simulink model "GCS"  (R2023a)
settings: Solver=FixedStepAuto  StartTime=0.0  StopTime=inf  FixedStep=1/100  RelTol=1e-3
undefined symbols (not defined in the file or in its folder): ARMED, AUX1, AUX2, f, MODE, NULL, Payload, Pitch, Roll, Throttle, Yaw
libraries: uavmavlinklib x3, vrlib x3, instrumentlib x2, instrumentseriallib x2, slrealtimeiplib x2, aerolibanimutils x1
settings Model: Creator=amc0121  LastModifiedBy=thesa
settings DebuggingCC: UnconnectedInputMsg=warning  UnconnectedOutputMsg=warning  UnconnectedLineMsg=warning
settings ModelReferenceCC: EnableRefExpFcnMdlSchedulingChecks=on
settings RTWCC: DLArmComputeVersion=19.05

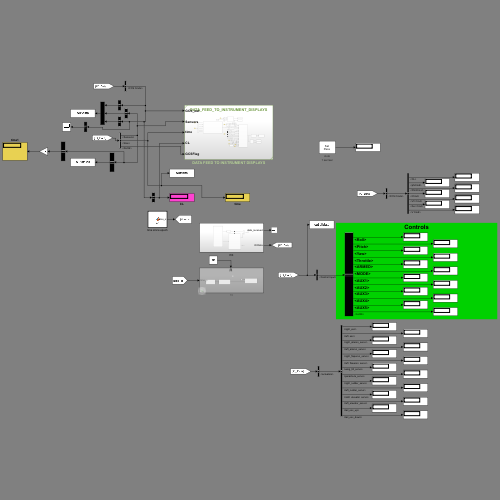
[thumbnail: Simulink's stored preview of the top-level diagram]
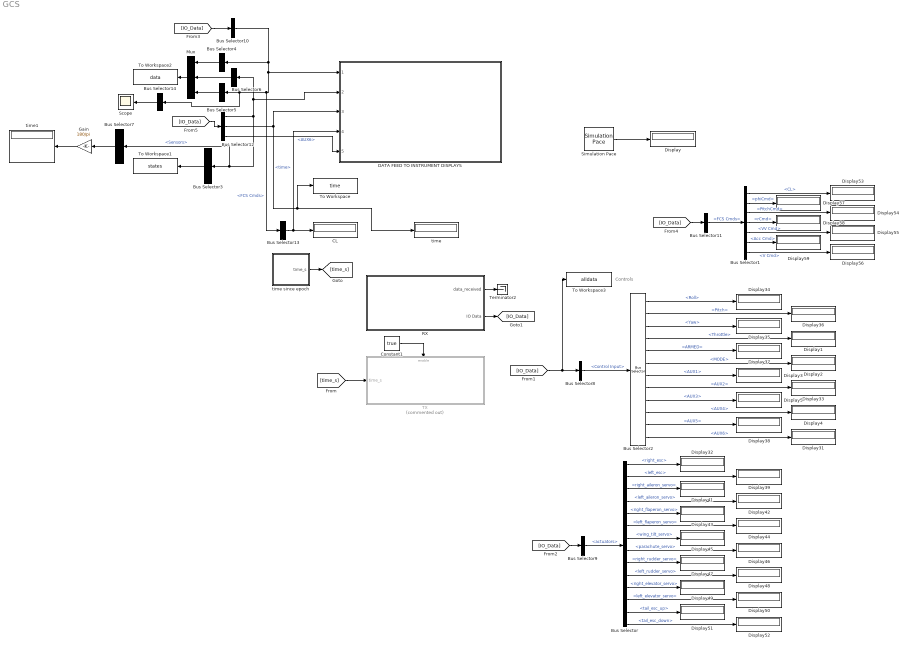
== system GCS ==
  note: Controls
  Bus Selector : BusSelector  OutputSignals=right_esc,left_esc,right_aileron_servo,left_aileron_servo,right_flaperon_servo,left_flaperon_servo,wing_tilt_servo,parachute_servo,right_rudder_servo,left_rudder_servo,right_elevator_servo,left_elevator_servo,tail_esc_up,tail_esc_down
  Bus Selector1 : BusSelector  OutputSignals=CL,CMDS.phiCmd,CMDS.PitchCmd,CMDS.rCmd,CMDS.VV Cmd,CMDS.Acc Cmd,CMDS.V Cmd
  Bus Selector10 : BusSelector  OutputSignals=Simulink Outputs.FCS Cmds
  Bus Selector11 : BusSelector  OutputSignals=Simulink Outputs.FCS Cmds
  Bus Selector12 : BusSelector  OutputSignals=Simulink Outputs.Sensors,Simulink Outputs.time,PX4/Simulink IO messages.sm_inbound_parsed.Control Input.AUX6
  Bus Selector13 : BusSelector  OutputSignals=CL  OutputAsBus=on
  Bus Selector14 : BusSelector  OutputSignals=PI.dlat  OutputAsBus=on
  Bus Selector2 : BusSelector  OutputSignals=Roll,Pitch,Yaw,Throttle,ARMED,MODE,AUX1,AUX2,AUX3,AUX4,AUX5,AUX6
  Bus Selector3 : BusSelector  OutputSignals=phi,theta,psi,p,q,r,TRK  OutputAsBus=on
  Bus Selector4 : BusSelector  OutputSignals=EMF,RPM,CMDS,TCS,PII,AP,GUIDANCE,NAV  OutputAsBus=on
  Bus Selector5 : BusSelector  OutputSignals=PI,CL  OutputAsBus=on
  Bus Selector6 : BusSelector  OutputSignals=VN,VE,hAGL,EAS,VFRD,VLAT,Lat,Long,VV,GC Flag,eph  OutputAsBus=on
  Bus Selector7 : BusSelector  OutputSignals=phi,theta,psi  OutputAsBus=on
  Bus Selector8 : BusSelector  OutputSignals=Simulink Inputs.Control Input
  Bus Selector9 : BusSelector  OutputSignals=Simulink Outputs.actuators
  CL : Display
  Constant1 : Constant  Value=true  OutDataTypeStr=boolean
  DATA FEED TO INSTRUMENT DISPLAYS : Subsystem  ReferencedSubsystem=DATA_FEED_TO_INSTRUMENT_DISPLAYS
  Display{,1..5,31..39,41..59} (34 alike) : Display
  Gain : Gain  Gain=180/pi
  Mux : Mux  Inputs=3
  RX : Subsystem
  Scope : Scope
  Simulation Pace : aerolibanimutils/Simulation Pace  SimulationPace=1  SleepMode=Auto  OutputPaceError=on  SampleTime=1/100
  TX : Subsystem  Commented=on  TreatAsAtomicUnit=on
  Terminator2 : Terminator
  To Workspace : ToWorkspace  VariableName=time  SampleTime=0.1
      settings: Save2DSignal=2-D array (concatenate along first dimension)
  To Workspace1 : ToWorkspace  VariableName=states  SampleTime=0.1
      settings: Save2DSignal=2-D array (concatenate along first dimension)
  To Workspace2 : ToWorkspace  VariableName=data  SampleTime=0.1
      settings: Save2DSignal=2-D array (concatenate along first dimension)
  To Workspace3 : ToWorkspace  VariableName=alldata  SaveFormat=Timeseries  SampleTime=-1
  time : Display
  time since epoch : MATLAB Function  TreatAsAtomicUnit=on
  time1 : Display
  wires:
  Bus Selector2/2 -> Display36/1  "<Pitch>"
  Bus Selector2/4 -> Display1/1  "<Throttle>"
  Bus Selector2/6 -> Display2/1  "<MODE>"
  Bus Selector2/8 -> Display33/1  "<AUX2>"
  Bus Selector2/1 -> Display34/1  "<Roll>"
  Bus Selector2/3 -> Display35/1  "<Yaw>"
  Bus Selector2/5 -> Display37/1  "<ARMED>"
  Bus Selector2/7 -> Display3/1  "<AUX1>"
  Bus Selector2/9 -> Display5/1  "<AUX3>"
  Bus Selector2/10 -> Display4/1  "<AUX4>"
  Bus Selector2/11 -> Display38/1  "<AUX5>"
  Simulation Pace/1 -> Display/1
  Bus Selector8/1 -> Bus Selector2/1  "<Control Input>"
  Bus Selector2/12 -> Display31/1  "<AUX6>"
  Bus Selector12/1 -> Bus Selector7/1, Bus Selector3/1, Bus Selector6/1, DATA FEED TO INSTRUMENT DISPLAYS/2  "<Sensors>"
  Bus Selector9/1 -> Bus Selector/1  "<actuators>"
  Bus Selector/1 -> Display32/1  "<right_esc>"
  Bus Selector/2 -> Display39/1  "<left_esc>"
  Bus Selector/3 -> Display41/1  "<right_aileron_servo>"
  Bus Selector/4 -> Display42/1  "<left_aileron_servo>"
  Bus Selector/5 -> Display43/1  "<right_flaperon_servo>"
  Bus Selector/6 -> Display44/1  "<left_flaperon_servo>"
  Bus Selector/7 -> Display45/1  "<wing_tilt_servo>"
  Bus Selector/8 -> Display46/1  "<parachute_servo>"
  Bus Selector/9 -> Display47/1  "<right_rudder_servo>"
  Bus Selector/10 -> Display48/1  "<left_rudder_servo>"
  Bus Selector/11 -> Display49/1  "<right_elevator_servo>"
  Bus Selector/12 -> Display50/1  "<left_elevator_servo>"
  Bus Selector/13 -> Display51/1  "<tail_esc_up>"
  Bus Selector/14 -> Display52/1  "<tail_esc_down>"
  Bus Selector10/1 -> Bus Selector13/1, Bus Selector14/1, Bus Selector5/1, DATA FEED TO INSTRUMENT DISPLAYS/1, Bus Selector4/1  "<FCS Cmds>"
  Bus Selector1/1 -> Display53/1  "<CL>"
  Bus Selector1/3 -> Display54/1  "<PitchCmd>"
  Bus Selector1/5 -> Display55/1  "<VV Cmd>"
  Bus Selector1/7 -> Display56/1  "<V Cmd>"
  Bus Selector1/2 -> Display57/1  "<phiCmd>"
  Bus Selector1/4 -> Display58/1  "<rCmd>"
  Bus Selector1/6 -> Display59/1  "<Acc Cmd>"
  RX/1(data_received) -> Terminator2/1
  time since epoch/1(time_s) -> [time_s]
  Constant1/1 -> TX/Enable
  [time_s] -> TX/1(time_s)
  Bus Selector12/2 -> DATA FEED TO INSTRUMENT DISPLAYS/3, To Workspace/1, time/1  "<time>"
  Bus Selector3/1 -> To Workspace1/1
  Bus Selector4/1 -> Mux/1
  Bus Selector5/1 -> Mux/3
  Mux/1 -> To Workspace2/1
  Bus Selector6/1 -> Mux/2
  Bus Selector7/1 -> Gain/1
  Gain/1 -> time1/1
  RX/2(IO Data) -> [IO_Data]
  [IO_Data] -> To Workspace3/1, Bus Selector8/1
  [IO_Data] -> Bus Selector9/1
  [IO_Data] -> Bus Selector10/1
  [IO_Data] -> Bus Selector11/1
  Bus Selector11/1 -> Bus Selector1/1  "<FCS Cmds>"
  [IO_Data] -> Bus Selector12/1
  Bus Selector13/1 -> DATA FEED TO INSTRUMENT DISPLAYS/4, CL/1
  Bus Selector14/1 -> Scope/1
  Bus Selector12/3 -> DATA FEED TO INSTRUMENT DISPLAYS/5  "<AUX6>"

== system GCS/RX ==
  AND : Logic  IconShape=distinctive  AllPortsSameDT=off  OutDataTypeStr=boolean
  Data Type Conversion : DataTypeConversion  OutDataTypeStr=boolean  SaturateOnIntegerOverflow=off  RndMeth=Floor
  Enabled Subsystem : Subsystem  TreatAsAtomicUnit=on
  Receiver Option : Subsystem  Variant=on  VariantControlMode=label  VariantControl=Choice  LabelModeActiveChoice=Choice_1
  data_received : Outport
  IO Data : Outport  Port=2
  wires:
  Receiver Option/1(Status) -> Data Type Conversion/1
  Data Type Conversion/1 -> Enabled Subsystem/Enable, AND/1
  Receiver Option/2(Data) -> Enabled Subsystem/1(ByteStream)
  Enabled Subsystem/1(data_received) -> AND/2
  AND/1 -> data_received/1
  Enabled Subsystem/2(IO Data) -> IO Data/1

== system GCS/TX ==
  time_s : Inport
  Enable : EnablePort
  Pilot Input Interpreter : Subsystem
  Raw Pilot Input : Subsystem
  SEND : Subsystem
  wires:
  time_s/1 -> SEND/1(time_s)
  Raw Pilot Input/1(Raw Pilot Input) -> Pilot Input Interpreter/1(Raw Pilot Input)
  Pilot Input Interpreter/1(Control Inputs) -> SEND/2(Control Inputs)

== system GCS/RX/Enabled Subsystem ==
  ByteStream : Inport
  Enable : EnablePort
  Data Type Conversion : DataTypeConversion  OutDataTypeStr=boolean  SaturateOnIntegerOverflow=off  RndMeth=Floor
  Enabled Subsystem : Subsystem  TreatAsAtomicUnit=on
  MAVLink Deserializer : uavmavlinklib/MAVLink Deserializer  dialectSource=Select from standard MAVLink dialects  dialect=common.xml  dialectCustom=common.xml  version=2  messageType=DEBUG_FLOAT_ARRAY  inputDataLength=off  SystemIDFilter=off  systemID=1  ComponentIDFilter=off  componentID=1  queueMsg=off  queueMsgSize=50  dropNum=off
  data_received : Outport
  IO Data : Outport  Port=2
  wires:
  MAVLink Deserializer/1 -> Data Type Conversion/1  "status"
  ByteStream/1 -> MAVLink Deserializer/1
  Data Type Conversion/1 -> data_received/1, Enabled Subsystem/Enable
  MAVLink Deserializer/2 -> Enabled Subsystem/1(DEBUG_FLOAT_ARRAY)
  Enabled Subsystem/1(IO Data) -> IO Data/1

== system GCS/RX/Receiver Option ==
  UDP: KGC : Subsystem  VariantControl=Choice_1
  UDP: QGC : Subsystem  VariantControl=Choice
  Status : Outport
  Data : Outport  Port=2

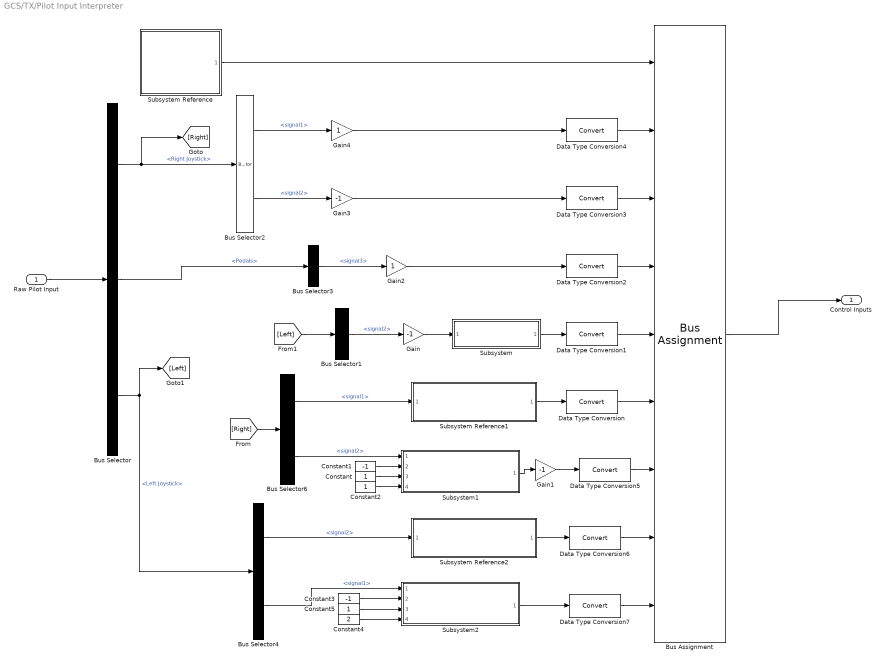
== system GCS/TX/Pilot Input Interpreter ==
  Raw Pilot Input : Inport
  Bus Assignment : BusAssignment  AssignedSignals=Roll,Pitch,Yaw,Throttle,ARMED,MODE,AUX1,AUX2
  Bus Selector : BusSelector  OutputSignals=Right Joystick,Pedals,Left Joystick
  Bus Selector1 : BusSelector  OutputSignals=Axes.signal2
  Bus Selector2 : BusSelector  OutputSignals=Axes.signal1,Axes.signal2
  Bus Selector3 : BusSelector  OutputSignals=Axes.signal3
  Bus Selector4 : BusSelector  OutputSignals=Buttons.signal2,Buttons.signal1
  Bus Selector6 : BusSelector  OutputSignals=Buttons.signal1,Buttons.signal2
  Constant : Constant
  Constant1 : Constant  Value=-1
  Constant2 : Constant
  Constant3 : Constant  Value=-1
  Constant4 : Constant  Value=2
  Constant5 : Constant
  Data Type Conversion{,1..7} (8 alike) : DataTypeConversion  SaturateOnIntegerOverflow=off  RndMeth=Floor
  Gain : Gain  Gain=-1
  Gain1 : Gain  Gain=-1
  Gain2 : Gain
  Gain3 : Gain  Gain=-1
  Gain4 : Gain
  Subsystem : Subsystem  ReferencedSubsystem=map_11_to_01
  Subsystem Reference : Subsystem  ReferencedSubsystem=sm_rc_initializer
  Subsystem Reference1 : Subsystem  ReferencedSubsystem=Push_button_to_Toggle_Switch
  Subsystem Reference2 : Subsystem  ReferencedSubsystem=Push_button_to_Toggle_Switch
  Subsystem1 : Subsystem  ReferencedSubsystem=Push_button_to_Rolling_Buffer
  Subsystem2 : Subsystem  ReferencedSubsystem=Push_button_to_Rolling_Buffer
  Control Inputs : Outport
  wires:
  Raw Pilot Input/1 -> Bus Selector/1
  Subsystem Reference/1 -> Bus Assignment/1
  Bus Assignment/1 -> Control Inputs/1
  Bus Selector6/1 -> Subsystem Reference1/1  "<signal1>"
  Bus Selector/3 -> [Left], Bus Selector4/1  "<Left Joystick>"
  Bus Selector1/1 -> Gain/1  "<signal2>"
  Bus Selector/1 -> [Right], Bus Selector2/1  "<Right Joystick>"
  Bus Selector2/2 -> Gain3/1  "<signal2>"
  Bus Selector/2 -> Bus Selector3/1  "<Pedals>"
  Bus Selector3/1 -> Gain2/1  "<signal3>"
  Data Type Conversion/1 -> Bus Assignment/6
  Data Type Conversion1/1 -> Bus Assignment/5
  Data Type Conversion2/1 -> Bus Assignment/4
  Data Type Conversion3/1 -> Bus Assignment/3
  Data Type Conversion4/1 -> Bus Assignment/2
  Data Type Conversion5/1 -> Bus Assignment/7
  Subsystem/1 -> Data Type Conversion1/1
  Gain/1 -> Subsystem/1
  Gain2/1 -> Data Type Conversion2/1
  Gain3/1 -> Data Type Conversion3/1
  Gain4/1 -> Data Type Conversion4/1
  Subsystem Reference1/1 -> Data Type Conversion/1
  Constant/1 -> Subsystem1/3
  Bus Selector6/2 -> Subsystem1/1  "<signal2>"
  Constant1/1 -> Subsystem1/2
  Data Type Conversion6/1 -> Bus Assignment/8
  Subsystem Reference2/1 -> Data Type Conversion6/1
  Bus Selector4/1 -> Subsystem Reference2/1  "<signal2>"
  Bus Selector2/1 -> Gain4/1  "<signal1>"
  [Left] -> Bus Selector1/1
  [Right] -> Bus Selector6/1
  Subsystem1/1 -> Gain1/1
  Data Type Conversion7/1 -> Bus Assignment/9
  Subsystem2/1 -> Data Type Conversion7/1
  Bus Selector4/2 -> Subsystem2/1  "<signal1>"
  Constant3/1 -> Subsystem2/2
  Constant5/1 -> Subsystem2/3
  Gain1/1 -> Data Type Conversion5/1
  Constant2/1 -> Subsystem1/4
  Constant4/1 -> Subsystem2/4

== system GCS/TX/Raw Pilot Input ==
  Bus Creator : BusCreator  Inputs=4
  Bus Creator1 : BusCreator  Inputs=1
  Subsystem1 : Subsystem
  Subsystem2 : Subsystem
  Subsystem3 : Subsystem
  T : Constant
  Raw Pilot Input : Outport
  wires:
  Subsystem3/1(Right Joystick) -> Bus Creator/2  "Right Joystick"
  Subsystem2/1(Left Joystick) -> Bus Creator/1  "Left Joystick"
  Bus Creator/1 -> Raw Pilot Input/1  "Raw Pilot Input"
  Subsystem1/1(Pedals) -> Bus Creator/3  "Pedals"
  T/1 -> Bus Creator1/1  "takeoff"
  Bus Creator1/1 -> Bus Creator/4  "GCS Displays"

== system GCS/TX/SEND ==
  time_s : Inport
  Control Inputs : Inport  Port=2
  DATA PACKING : Subsystem
  Rate Transition : RateTransition  OutPortSampleTime=1/20
  Send Option : Subsystem  Variant=on  VariantControlMode=label  VariantControl=Choice  LabelModeActiveChoice=Choice_2
  wires:
  Control Inputs/1 -> DATA PACKING/2(Control Inputs)
  time_s/1 -> DATA PACKING/1(time_s)
  DATA PACKING/1(data) -> Rate Transition/1
  Rate Transition/1 -> Send Option/1(data)

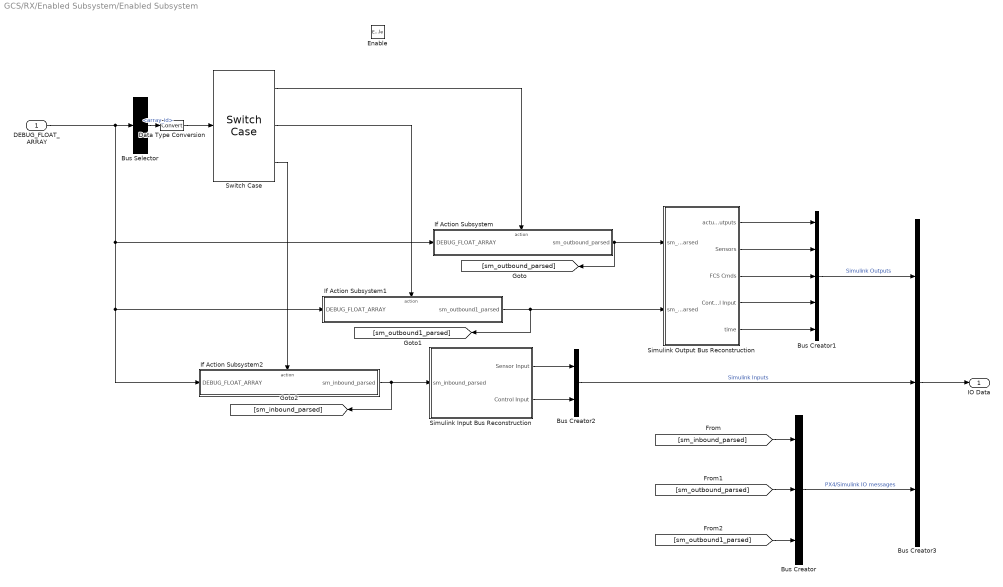
== system GCS/RX/Enabled Subsystem/Enabled Subsystem ==
  DEBUG_FLOAT_ARRAY : Inport
  Enable : EnablePort
  Bus Creator : BusCreator  Inputs=3
  Bus Creator1 : BusCreator  Inputs=5
  Bus Creator2 : BusCreator  Inputs=2
  Bus Creator3 : BusCreator  Inputs=3
  Bus Selector : BusSelector  OutputSignals=Payload.array_id
  Data Type Conversion : DataTypeConversion  SaturateOnIntegerOverflow=off  RndMeth=Floor
  If Action Subsystem : Subsystem  TreatAsAtomicUnit=on
  If Action Subsystem1 : Subsystem  TreatAsAtomicUnit=on
  If Action Subsystem2 : Subsystem  TreatAsAtomicUnit=on
  Simulink Input Bus Reconstruction : Subsystem
  Simulink Output Bus Reconstruction : Subsystem
  Switch Case : SwitchCase  CaseConditions="{100,  101, 200}"  ShowDefaultCase=off
  IO Data : Outport
  wires:
  DEBUG_FLOAT_ARRAY/1 -> Bus Selector/1, If Action Subsystem/1(DEBUG_FLOAT_ARRAY), If Action Subsystem2/1(DEBUG_FLOAT_ARRAY), If Action Subsystem1/1(DEBUG_FLOAT_ARRAY)
  Bus Selector/1 -> Data Type Conversion/1  "<array_id>"
  Switch Case/1 -> If Action Subsystem/Action
  Switch Case/2 -> If Action Subsystem1/Action
  If Action Subsystem/1(sm_outbound_parsed) -> [sm_outbound_parsed], Simulink Output Bus Reconstruction/1(sm_outbound_parsed)
  If Action Subsystem1/1(sm_outbound1_parsed) -> [sm_outbound1_parsed], Simulink Output Bus Reconstruction/2(sm_outbound1_parsed)
  Simulink Output Bus Reconstruction/1(actuator_outputs) -> Bus Creator1/1
  Simulink Output Bus Reconstruction/2(Sensors) -> Bus Creator1/2
  Simulink Output Bus Reconstruction/3(FCS Cmds) -> Bus Creator1/3
  Switch Case/3 -> If Action Subsystem2/Action
  If Action Subsystem2/1(sm_inbound_parsed) -> [sm_inbound_parsed], Simulink Input Bus Reconstruction/1(sm_inbound_parsed)
  Simulink Input Bus Reconstruction/1(Sensor Input) -> Bus Creator2/1
  Simulink Input Bus Reconstruction/2(Control Input) -> Bus Creator2/2
  Data Type Conversion/1 -> Switch Case/1
  Simulink Output Bus Reconstruction/4(Control Input) -> Bus Creator1/4
  Simulink Output Bus Reconstruction/5(time) -> Bus Creator1/5
  Bus Creator1/1 -> Bus Creator3/1  "Simulink Outputs"
  Bus Creator2/1 -> Bus Creator3/2  "Simulink Inputs"
  Bus Creator/1 -> Bus Creator3/3  "PX4/Simulink IO messages"
  [sm_inbound_parsed] -> Bus Creator/1
  [sm_outbound_parsed] -> Bus Creator/2
  [sm_outbound1_parsed] -> Bus Creator/3
  Bus Creator3/1 -> IO Data/1

== system GCS/RX/Receiver Option/UDP: KGC ==
  QGC : instrumentlib/UDP Receive  LocalAddress=127.0.0.1  LocalPort=14750  EnablePortSharing=off  Host=localhost  Port=14751  GetLatestData=off  DataSize=256  DataType=uint8  ASCIIFormatting=%f,  Terminator=LF  CustomTerminator=10  ByteOrder=big-endian  EnableBlockingMode=off  Timeout=100  SampleTime=1/100  SimulateUsing=Interpreted execution
  Data : Outport
  Status : Outport  Port=2
  wires:
  QGC/2 -> Status/1
  QGC/1 -> Data/1

== system GCS/RX/Receiver Option/UDP: QGC ==
  QGC : instrumentlib/UDP Receive  LocalAddress=127.0.0.1  LocalPort=14445  EnablePortSharing=off  Host=localhost  Port=9090  GetLatestData=off  DataSize=96  DataType=uint8  ASCIIFormatting=%f,  Terminator=LF  CustomTerminator=10  ByteOrder=big-endian  EnableBlockingMode=off  Timeout=100  SampleTime=1/100  SimulateUsing=Interpreted execution
  Data : Outport
  Status : Outport  Port=2
  wires:
  QGC/1 -> Data/1
  QGC/2 -> Status/1

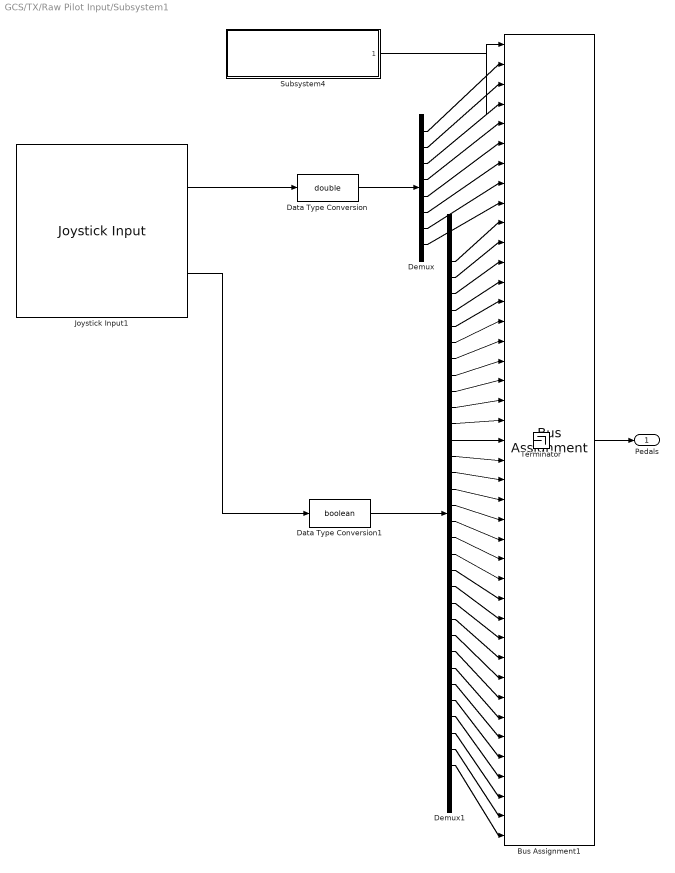
== system GCS/TX/Raw Pilot Input/Subsystem1 ==
  Bus Assignment1 : BusAssignment  AssignedSignals=Axes.signal1,Axes.signal2,Axes.signal3,Axes.signal4,Axes.signal5,Axes.signal6,Axes.signal7,Axes.signal8,Buttons.signal1,Buttons.signal2,Buttons.signal3,Buttons.signal4,Buttons.signal5,Buttons.signal6,Buttons.signal7,Buttons.signal8,Buttons.signal9,Buttons.signal10,Buttons.signal11,Buttons.signal12,Buttons.signal13,Buttons.signal14,Buttons.signal15,Buttons.signal16,Buttons.signal17,Buttons.signal18,Buttons.signal19,Buttons.signal20,Buttons.signal21,Buttons.signal22,Buttons.signal23,Buttons.signal24,Buttons.signal25,Buttons.signal26,Buttons.signal27,Buttons.signal28,Buttons.signal29,Buttons.signal30,Buttons.signal31,Buttons.signal32
  Data Type Conversion : DataTypeConversion  OutDataTypeStr=double  SaturateOnIntegerOverflow=off  RndMeth=Floor
  Data Type Conversion1 : DataTypeConversion  OutDataTypeStr=boolean  SaturateOnIntegerOverflow=off  RndMeth=Floor
  Demux : Demux  Outputs=8
  Demux1 : Demux  Outputs=32
  Joystick Input1 : vrlib/Joystick Input  joyid=3  adjustports=off  forcefeed=off
  Subsystem4 : Subsystem  ReferencedSubsystem=JoystickInitializer
  Terminator : Terminator
  Pedals : Outport
  wires:
  Demux1/1 -> Bus Assignment1/10
  Demux1/12 -> Bus Assignment1/21
  Demux1/8 -> Bus Assignment1/17
  Demux1/17 -> Bus Assignment1/26
  Demux1/16 -> Bus Assignment1/25
  Demux1/3 -> Bus Assignment1/12
  Demux1/10 -> Bus Assignment1/19
  Bus Assignment1/1 -> Pedals/1
  Demux1/15 -> Bus Assignment1/24
  Joystick Input1/2 -> Data Type Conversion1/1
  Demux1/11 -> Bus Assignment1/20
  Demux/1 -> Bus Assignment1/2
  Demux1/13 -> Bus Assignment1/22
  Demux1/19 -> Bus Assignment1/28
  Demux1/2 -> Bus Assignment1/11
  Demux1/6 -> Bus Assignment1/15
  Demux1/4 -> Bus Assignment1/13
  Demux1/18 -> Bus Assignment1/27
  Demux1/7 -> Bus Assignment1/16
  Demux1/14 -> Bus Assignment1/23
  Demux1/9 -> Bus Assignment1/18
  Joystick Input1/1 -> Data Type Conversion/1
  Demux1/5 -> Bus Assignment1/14
  Subsystem4/1 -> Bus Assignment1/1
  Demux/2 -> Bus Assignment1/3
  Demux/8 -> Bus Assignment1/9
  Demux/7 -> Bus Assignment1/8
  Demux/6 -> Bus Assignment1/7
  Demux/5 -> Bus Assignment1/6
  Demux/4 -> Bus Assignment1/5
  Demux/3 -> Bus Assignment1/4
  Demux1/20 -> Bus Assignment1/29
  Demux1/21 -> Bus Assignment1/30
  Demux1/22 -> Bus Assignment1/31
  Demux1/23 -> Bus Assignment1/32
  Demux1/24 -> Bus Assignment1/33
  Demux1/25 -> Bus Assignment1/34
  Demux1/26 -> Bus Assignment1/35
  Demux1/27 -> Bus Assignment1/36
  Demux1/28 -> Bus Assignment1/37
  Demux1/29 -> Bus Assignment1/38
  Demux1/30 -> Bus Assignment1/39
  Demux1/31 -> Bus Assignment1/40
  Demux1/32 -> Bus Assignment1/41
  Data Type Conversion/1 -> Demux/1
  Data Type Conversion1/1 -> Demux1/1

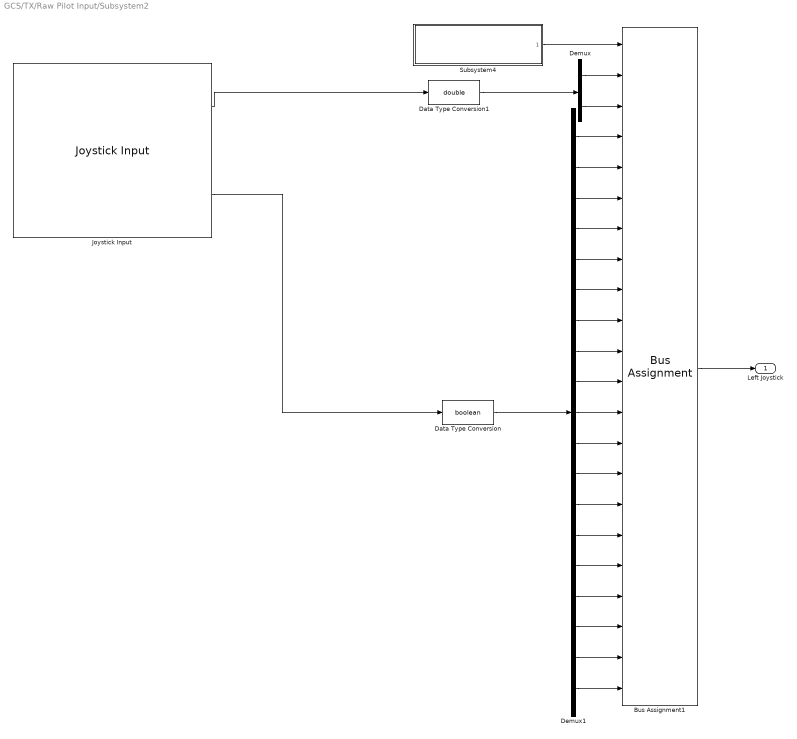
== system GCS/TX/Raw Pilot Input/Subsystem2 ==
  Bus Assignment1 : BusAssignment  AssignedSignals=Axes.signal1,Axes.signal2,Buttons.signal1,Buttons.signal2,Buttons.signal3,Buttons.signal4,Buttons.signal5,Buttons.signal6,Buttons.signal7,Buttons.signal8,Buttons.signal9,Buttons.signal10,Buttons.signal11,Buttons.signal12,Buttons.signal13,Buttons.signal14,Buttons.signal15,Buttons.signal16,Buttons.signal17,Buttons.signal18,Buttons.signal19
  Data Type Conversion : DataTypeConversion  OutDataTypeStr=boolean  SaturateOnIntegerOverflow=off  RndMeth=Floor
  Data Type Conversion1 : DataTypeConversion  OutDataTypeStr=double  SaturateOnIntegerOverflow=off  RndMeth=Floor
  Demux : Demux  Outputs=2
  Demux1 : Demux  Outputs=19
  Joystick Input : vrlib/Joystick Input  joyid=1  adjustports=on  forcefeed=off
  Subsystem4 : Subsystem  ReferencedSubsystem=JoystickInitializer
  Left Joystick : Outport
  wires:
  Demux/2 -> Bus Assignment1/3
  Subsystem4/1 -> Bus Assignment1/1
  Demux1/5 -> Bus Assignment1/8
  Demux1/9 -> Bus Assignment1/12
  Demux1/14 -> Bus Assignment1/17
  Demux1/7 -> Bus Assignment1/10
  Demux1/18 -> Bus Assignment1/21
  Demux1/4 -> Bus Assignment1/7
  Demux1/6 -> Bus Assignment1/9
  Demux1/2 -> Bus Assignment1/5
  Demux1/19 -> Bus Assignment1/22
  Demux1/13 -> Bus Assignment1/16
  Demux/1 -> Bus Assignment1/2
  Demux1/11 -> Bus Assignment1/14
  Demux1/15 -> Bus Assignment1/18
  Bus Assignment1/1 -> Left Joystick/1
  Demux1/10 -> Bus Assignment1/13
  Demux1/3 -> Bus Assignment1/6
  Demux1/16 -> Bus Assignment1/19
  Demux1/17 -> Bus Assignment1/20
  Demux1/8 -> Bus Assignment1/11
  Demux1/12 -> Bus Assignment1/15
  Demux1/1 -> Bus Assignment1/4
  Joystick Input/1 -> Data Type Conversion1/1
  Joystick Input/2 -> Data Type Conversion/1
  Data Type Conversion/1 -> Demux1/1
  Data Type Conversion1/1 -> Demux/1

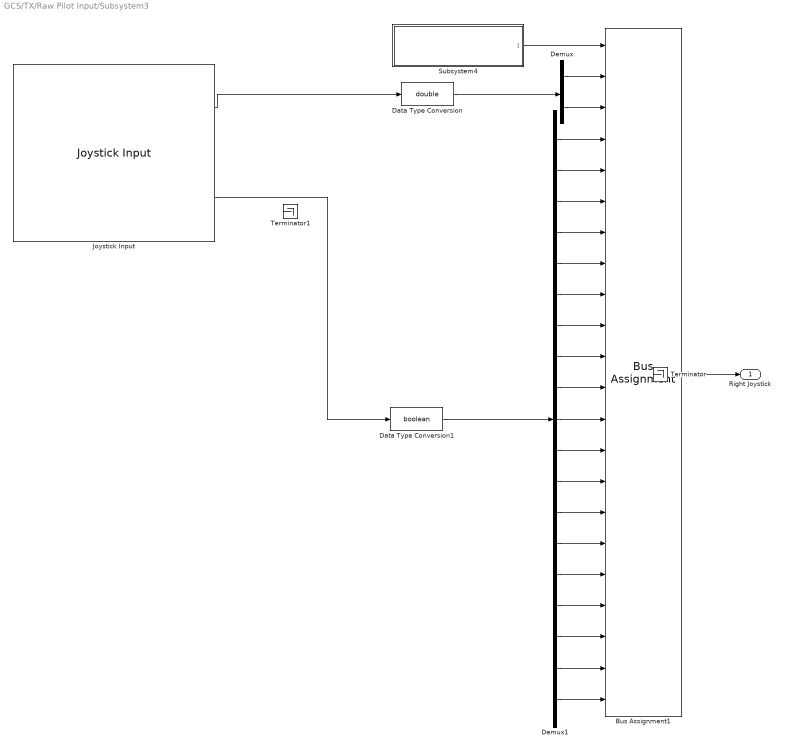
== system GCS/TX/Raw Pilot Input/Subsystem3 ==
  Bus Assignment1 : BusAssignment  AssignedSignals=Axes.signal1,Axes.signal2,Buttons.signal1,Buttons.signal2,Buttons.signal3,Buttons.signal4,Buttons.signal5,Buttons.signal6,Buttons.signal7,Buttons.signal8,Buttons.signal9,Buttons.signal10,Buttons.signal11,Buttons.signal12,Buttons.signal13,Buttons.signal14,Buttons.signal15,Buttons.signal16,Buttons.signal17,Buttons.signal18,Buttons.signal19
  Data Type Conversion : DataTypeConversion  OutDataTypeStr=double  SaturateOnIntegerOverflow=off  RndMeth=Floor
  Data Type Conversion1 : DataTypeConversion  OutDataTypeStr=boolean  SaturateOnIntegerOverflow=off  RndMeth=Floor
  Demux : Demux  Outputs=2
  Demux1 : Demux  Outputs=19
  Joystick Input : vrlib/Joystick Input  joyid=2  adjustports=on  forcefeed=off
  Subsystem4 : Subsystem  ReferencedSubsystem=JoystickInitializer
  Terminator : Terminator
  Terminator1 : Terminator
  Right Joystick : Outport
  wires:
  Demux1/1 -> Bus Assignment1/4
  Demux1/12 -> Bus Assignment1/15
  Demux1/8 -> Bus Assignment1/11
  Demux1/17 -> Bus Assignment1/20
  Demux1/16 -> Bus Assignment1/19
  ? -> Terminator1/1
  Demux1/3 -> Bus Assignment1/6
  Demux1/10 -> Bus Assignment1/13
  Bus Assignment1/1 -> Right Joystick/1
  Demux1/15 -> Bus Assignment1/18
  Joystick Input/2 -> Data Type Conversion1/1
  Demux1/11 -> Bus Assignment1/14
  Demux/1 -> Bus Assignment1/2
  Demux1/13 -> Bus Assignment1/16
  Demux1/19 -> Bus Assignment1/22
  Demux1/2 -> Bus Assignment1/5
  Demux1/6 -> Bus Assignment1/9
  Demux1/4 -> Bus Assignment1/7
  Demux1/18 -> Bus Assignment1/21
  Demux1/7 -> Bus Assignment1/10
  Demux1/14 -> Bus Assignment1/17
  Demux1/9 -> Bus Assignment1/12
  Joystick Input/1 -> Data Type Conversion/1
  Demux1/5 -> Bus Assignment1/8
  Subsystem4/1 -> Bus Assignment1/1
  Demux/2 -> Bus Assignment1/3
  Data Type Conversion/1 -> Demux/1
  Data Type Conversion1/1 -> Demux1/1

== system GCS/TX/SEND/DATA PACKING ==
  time_s : Inport
  Control Inputs : Inport  Port=2
  Bus Creator : BusCreator  Inputs=2
  SIMULINK INBOUND CONTROL : Subsystem
  data : Outport
  wires:
  SIMULINK INBOUND CONTROL/1(data) -> Bus Creator/1  "data"
  Control Inputs/1 -> SIMULINK INBOUND CONTROL/2(Control Inputs)
  time_s/1 -> SIMULINK INBOUND CONTROL/1(time_s)
  SIMULINK INBOUND CONTROL/2(length) -> Bus Creator/2  "length"
  Bus Creator/1 -> data/1

== system GCS/TX/SEND/Send Option ==
  data : Inport
  Serial : Subsystem  VariantControl=Choice_1
  UDP KGC : Subsystem  VariantControl=Choice_2
  UDP QGC : Subsystem  VariantControl=Choice

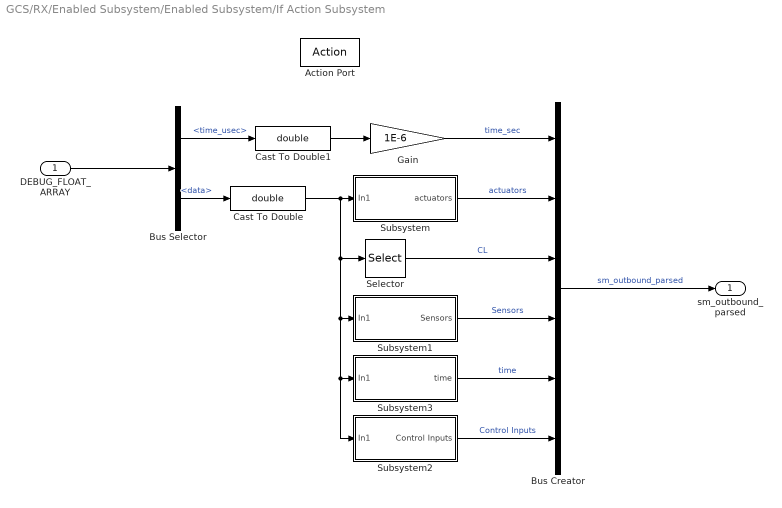
== system GCS/RX/Enabled Subsystem/Enabled Subsystem/If Action Subsystem ==
  DEBUG_FLOAT_ARRAY : Inport
  Action Port : ActionPort  ActionPortLabel=case [ 100 ]:
  Bus Creator : BusCreator  Inputs=6
  Bus Selector : BusSelector  OutputSignals=Payload.time_usec,Payload.data
  Cast To Double : DataTypeConversion  OutDataTypeStr=double  SaturateOnIntegerOverflow=off  RndMeth=Floor
  Cast To Double1 : DataTypeConversion  OutDataTypeStr=double  SaturateOnIntegerOverflow=off  RndMeth=Floor
  Gain : Gain  Gain=1E-6
  Selector : Selector  InputPortWidth=58  IndexOptions=Index vector (dialog)  Indices=[17]  OutputSizes=1
  Subsystem : Subsystem
  Subsystem1 : Subsystem
  Subsystem2 : Subsystem
  Subsystem3 : Subsystem
  sm_outbound_parsed : Outport
  wires:
  Cast To Double/1 -> Subsystem2/1(In1), Subsystem3/1(In1), Subsystem1/1(In1), Selector/1, Subsystem/1(In1)
  Gain/1 -> Bus Creator/1  "time_sec"
  Cast To Double1/1 -> Gain/1
  Subsystem/1(actuators) -> Bus Creator/2  "actuators"
  DEBUG_FLOAT_ARRAY/1 -> Bus Selector/1
  Selector/1 -> Bus Creator/3  "CL"
  Bus Creator/1 -> sm_outbound_parsed/1  "sm_outbound_parsed"
  Bus Selector/2 -> Cast To Double/1  "<data>"
  Bus Selector/1 -> Cast To Double1/1  "<time_usec>"
  Subsystem1/1(Sensors) -> Bus Creator/4  "Sensors"
  Subsystem2/1(Control Inputs) -> Bus Creator/6  "Control Inputs"
  Subsystem3/1(time) -> Bus Creator/5  "time"

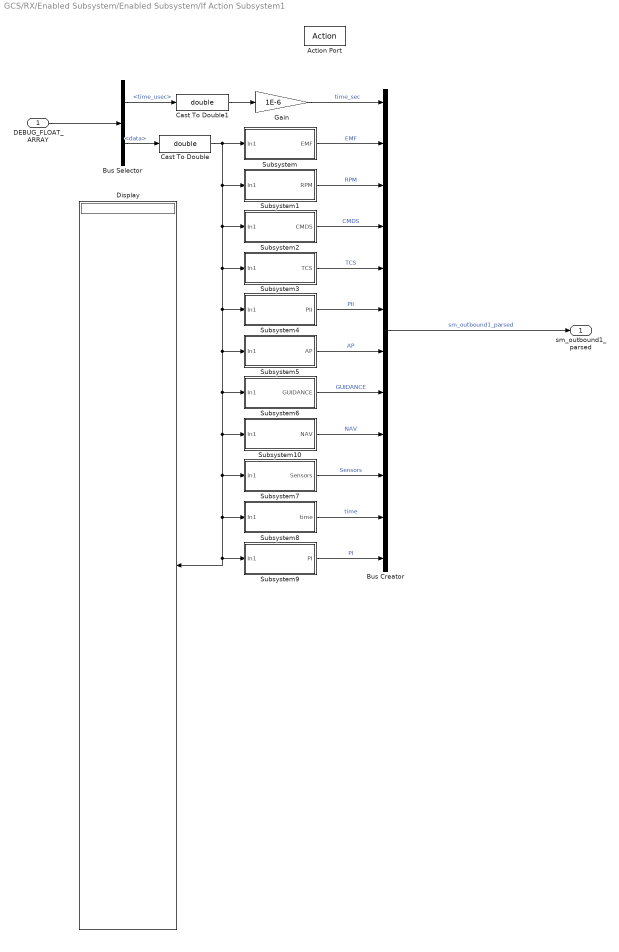
== system GCS/RX/Enabled Subsystem/Enabled Subsystem/If Action Subsystem1 ==
  DEBUG_FLOAT_ARRAY : Inport
  Action Port : ActionPort  ActionPortLabel=case [ 101 ]:
  Bus Creator : BusCreator  Inputs=12
  Bus Selector : BusSelector  OutputSignals=Payload.time_usec,Payload.data
  Cast To Double : DataTypeConversion  OutDataTypeStr=double  SaturateOnIntegerOverflow=off  RndMeth=Floor
  Cast To Double1 : DataTypeConversion  OutDataTypeStr=double  SaturateOnIntegerOverflow=off  RndMeth=Floor
  Display : Display
  Gain : Gain  Gain=1E-6
  Subsystem : Subsystem
  Subsystem1 : Subsystem
  Subsystem10 : Subsystem
  Subsystem2 : Subsystem
  Subsystem3 : Subsystem
  Subsystem4 : Subsystem
  Subsystem5 : Subsystem
  Subsystem6 : Subsystem
  Subsystem7 : Subsystem
  Subsystem8 : Subsystem
  Subsystem9 : Subsystem
  sm_outbound1_parsed : Outport
  wires:
  Subsystem10/1(NAV) -> Bus Creator/9  "NAV"
  Subsystem8/1(time) -> Bus Creator/11  "time"
  Subsystem4/1(PII) -> Bus Creator/6  "PII"
  Subsystem5/1(AP) -> Bus Creator/7  "AP"
  Subsystem7/1(Sensors) -> Bus Creator/10  "Sensors"
  Subsystem9/1(PI) -> Bus Creator/12  "PI"
  Gain/1 -> Bus Creator/1  "time_sec"
  Subsystem6/1(GUIDANCE) -> Bus Creator/8  "GUIDANCE"
  Subsystem1/1(RPM) -> Bus Creator/3  "RPM"
  Cast To Double/1 -> Subsystem/1(In1), Display/1, Subsystem9/1(In1), Subsystem8/1(In1), Subsystem7/1(In1), Subsystem10/1(In1), Subsystem6/1(In1), Subsystem5/1(In1), Subsystem4/1(In1), Subsystem3/1(In1), Subsystem2/1(In1), Subsystem1/1(In1)
  DEBUG_FLOAT_ARRAY/1 -> Bus Selector/1
  Subsystem2/1(CMDS) -> Bus Creator/4  "CMDS"
  Bus Selector/1 -> Cast To Double1/1  "<time_usec>"
  Cast To Double1/1 -> Gain/1
  Bus Selector/2 -> Cast To Double/1  "<data>"
  Subsystem/1(EMF) -> Bus Creator/2  "EMF"
  Bus Creator/1 -> sm_outbound1_parsed/1  "sm_outbound1_parsed"
  Subsystem3/1(TCS) -> Bus Creator/5  "TCS"

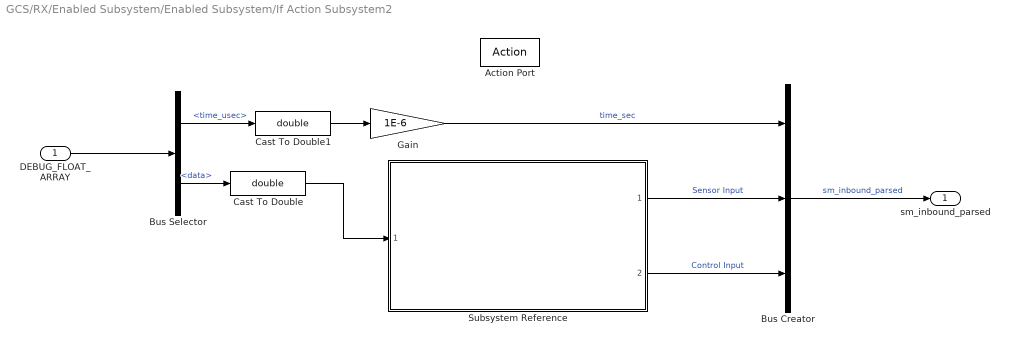
== system GCS/RX/Enabled Subsystem/Enabled Subsystem/If Action Subsystem2 ==
  DEBUG_FLOAT_ARRAY : Inport
  Action Port : ActionPort  ActionPortLabel=case [ 200 ]:
  Bus Creator : BusCreator  Inputs=3
  Bus Selector : BusSelector  OutputSignals=Payload.time_usec,Payload.data
  Cast To Double : DataTypeConversion  OutDataTypeStr=double  SaturateOnIntegerOverflow=off  RndMeth=Floor
  Cast To Double1 : DataTypeConversion  OutDataTypeStr=double  SaturateOnIntegerOverflow=off  RndMeth=Floor
  Gain : Gain  Gain=1E-6
  Subsystem Reference : Subsystem  ReferencedSubsystem=sm_inbound_interpreter
  sm_inbound_parsed : Outport
  wires:
  Bus Creator/1 -> sm_inbound_parsed/1  "sm_inbound_parsed"
  Subsystem Reference/2 -> Bus Creator/3  "Control Input"
  Gain/1 -> Bus Creator/1  "time_sec"
  Cast To Double1/1 -> Gain/1
  Subsystem Reference/1 -> Bus Creator/2  "Sensor Input"
  Cast To Double/1 -> Subsystem Reference/1
  DEBUG_FLOAT_ARRAY/1 -> Bus Selector/1
  Bus Selector/2 -> Cast To Double/1  "<data>"
  Bus Selector/1 -> Cast To Double1/1  "<time_usec>"

== system GCS/RX/Enabled Subsystem/Enabled Subsystem/Simulink Input Bus Reconstruction ==
  sm_inbound_parsed : Inport
  Bus Selector : BusSelector  OutputSignals=Sensor Input,Control Input
  Sensor Input : Outport
  Control Input : Outport  Port=2
  wires:
  sm_inbound_parsed/1 -> Bus Selector/1
  Bus Selector/1 -> Sensor Input/1  "<Sensor Input>"
  Bus Selector/2 -> Control Input/1  "<Control Input>"

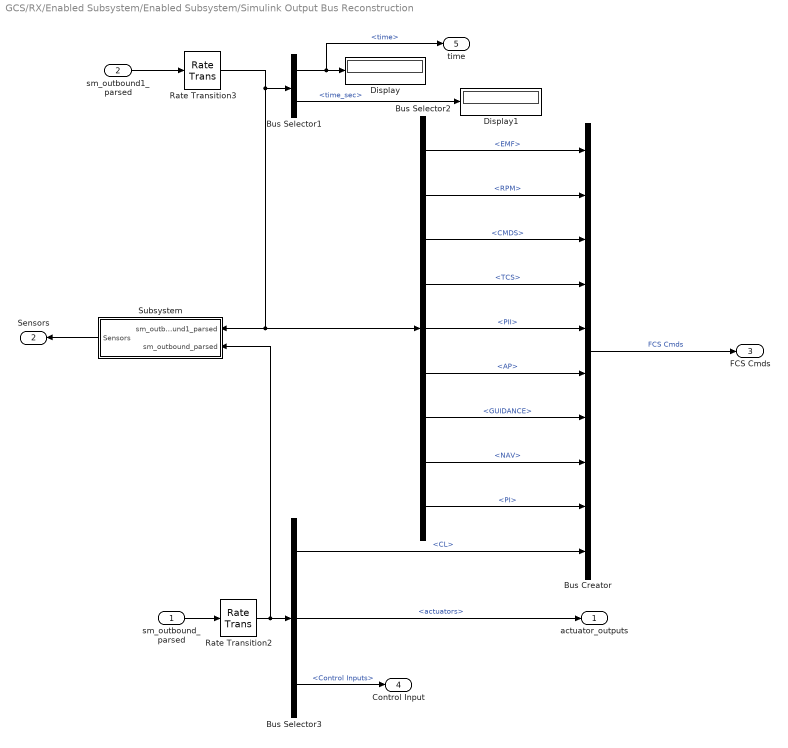
== system GCS/RX/Enabled Subsystem/Enabled Subsystem/Simulink Output Bus Reconstruction ==
  sm_outbound_parsed : Inport
  sm_outbound1_parsed : Inport  Port=2
  Bus Creator : BusCreator  Inputs=10
  Bus Selector1 : BusSelector  OutputSignals=time,time_sec
  Bus Selector2 : BusSelector  OutputSignals=EMF,RPM,CMDS,TCS,PII,AP,GUIDANCE,NAV,PI
  Bus Selector3 : BusSelector  OutputSignals=CL,actuators,Control Inputs
  Display : Display
  Display1 : Display
  Rate Transition2 : RateTransition  OutPortSampleTimeOpt=Inherit
  Rate Transition3 : RateTransition  OutPortSampleTimeOpt=Inherit
  Subsystem : Subsystem
  actuator_outputs : Outport
  Sensors : Outport  Port=2
  FCS Cmds : Outport  Port=3
  Control Input : Outport  Port=4
  time : Outport  Port=5
  wires:
  Bus Selector2/8 -> Bus Creator/8  "<NAV>"
  Bus Selector2/1 -> Bus Creator/1  "<EMF>"
  Bus Selector3/1 -> Bus Creator/10  "<CL>"
  Rate Transition3/1 -> Subsystem/1(sm_outbound1_parsed), Bus Selector2/1, Bus Selector1/1
  Bus Selector2/4 -> Bus Creator/4  "<TCS>"
  Bus Selector2/2 -> Bus Creator/2  "<RPM>"
  Bus Selector3/2 -> actuator_outputs/1  "<actuators>"
  Bus Selector2/3 -> Bus Creator/3  "<CMDS>"
  Bus Selector2/7 -> Bus Creator/7  "<GUIDANCE>"
  Rate Transition2/1 -> Subsystem/2(sm_outbound_parsed), Bus Selector3/1
  Bus Creator/1 -> FCS Cmds/1  "FCS Cmds"
  Bus Selector2/5 -> Bus Creator/5  "<PII>"
  Bus Selector2/6 -> Bus Creator/6  "<AP>"
  Bus Selector2/9 -> Bus Creator/9  "<PI>"
  sm_outbound_parsed/1 -> Rate Transition2/1
  sm_outbound1_parsed/1 -> Rate Transition3/1
  Bus Selector1/1 -> time/1, Display/1  "<time>"
  Bus Selector1/2 -> Display1/1  "<time_sec>"
  Subsystem/1(Sensors) -> Sensors/1
  Bus Selector3/3 -> Control Input/1  "<Control Inputs>"

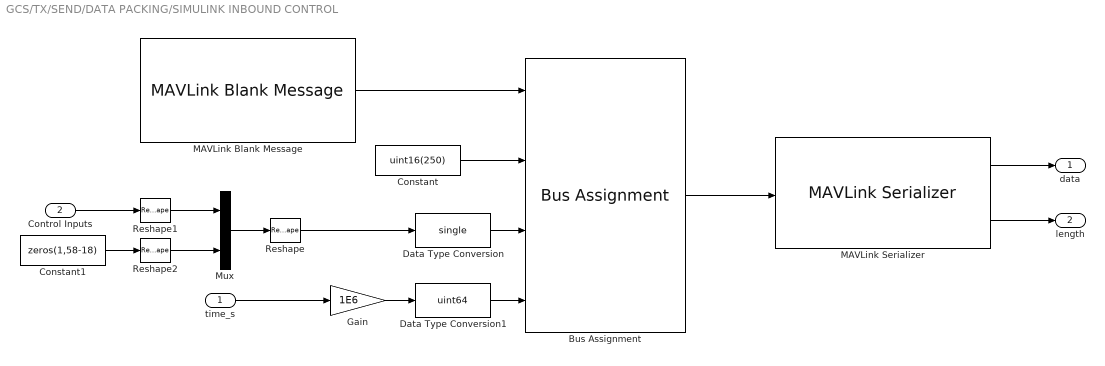
== system GCS/TX/SEND/DATA PACKING/SIMULINK INBOUND CONTROL ==
  time_s : Inport
  Control Inputs : Inport  Port=2
  Bus Assignment : BusAssignment  AssignedSignals=Payload.array_id,Payload.data,Payload.time_usec
  Constant : Constant  Value=uint16(250)  OutDataTypeStr=uint16
  Constant1 : Constant  Value=zeros(1,58-18)
  Data Type Conversion : DataTypeConversion  OutDataTypeStr=single  SaturateOnIntegerOverflow=off  RndMeth=Floor
  Data Type Conversion1 : DataTypeConversion  OutDataTypeStr=uint64  SaturateOnIntegerOverflow=off  RndMeth=Floor
  Gain : Gain  Gain=1E6
  MAVLink Blank Message : uavmavlinklib/MAVLink Blank Message  dialectSource=Select from standard MAVLink dialects  dialect=common.xml  dialectCustom=common.xml  version=2  messageType=DEBUG_FLOAT_ARRAY  SystemID=201  ComponentID=190  SampleTime=inf
  MAVLink Serializer : uavmavlinklib/MAVLink Serializer  dialectSource=Select from standard MAVLink dialects  dialect=common.xml  dialectCustom=common.xml  version=2  messageType=DEBUG_FLOAT_ARRAY
  Mux : Mux  Inputs=2
  Reshape : Reshape
  Reshape1 : Reshape
  Reshape2 : Reshape
  data : Outport
  length : Outport  Port=2
  wires:
  Bus Assignment/1 -> MAVLink Serializer/1
  MAVLink Blank Message/1 -> Bus Assignment/1
  MAVLink Serializer/2 -> length/1
  Constant/1 -> Bus Assignment/2
  MAVLink Serializer/1 -> data/1
  Control Inputs/1 -> Reshape1/1
  Reshape/1 -> Data Type Conversion/1
  Data Type Conversion/1 -> Bus Assignment/3
  time_s/1 -> Gain/1
  Gain/1 -> Data Type Conversion1/1
  Reshape1/1 -> Mux/1
  Reshape2/1 -> Mux/2
  Constant1/1 -> Reshape2/1
  Mux/1 -> Reshape/1
  Data Type Conversion1/1 -> Bus Assignment/4

== system GCS/TX/SEND/Send Option/Serial ==
  data : Inport
  Bus Selector : BusSelector  OutputSignals=data,length
  Data Type Conversion : DataTypeConversion  SaturateOnIntegerOverflow=off  RndMeth=Floor
  Serial Configuration : instrumentseriallib/Serial Configuration  Priority=-200000  PortSel=COM6  Port=COM6  ComPort=COM6  BaudRate=115200  DataBits=8  Parity=none  StopBits=1  ByteOrder=little-endian  FlowControl=none  Timeout=10  SimulateUsing=Interpreted execution  BlockInModel=on  aMode=1
      settings: LibrarySourceBlock=embeddedtargetslib/Host Communication/Serial Configuration
  Serial Send : instrumentseriallib/Serial Send  Priority=1  PortSel=COM6  Port=COM6  ComPort=COM6  Header=[]  Terminator=NULL ('\0')  CustomTerminator=[]  EnableBlockingMode=on  SimulateUsing=Interpreted execution  BlockInModel=on  aMode=1
      settings: LibrarySourceBlock=embeddedtargetslib/Host Communication/Serial Send
  Terminator : Terminator
  wires:
  Data Type Conversion/1 -> Terminator/1
  data/1 -> Bus Selector/1
  Bus Selector/1 -> Serial Send/1  "<data>"
  Bus Selector/2 -> Data Type Conversion/1  "<length>"

== system GCS/TX/SEND/Send Option/UDP KGC ==
  data : Inport
  Bus Selector1 : BusSelector  OutputSignals=data,length
  Data Type Conversion : DataTypeConversion  SaturateOnIntegerOverflow=off  RndMeth=Floor
  UDP : slrealtimeiplib/UDP Send  useHostTargetConn=on  toAddress=127.0.0.1  toPort=14651  sampleTime=-1  enableMessage=off  localPort=14650
  wires:
  data/1 -> Bus Selector1/1
  Bus Selector1/2 -> Data Type Conversion/1  "<length>"
  Data Type Conversion/1 -> UDP/2
  Bus Selector1/1 -> UDP/1  "<data>"

== system GCS/TX/SEND/Send Option/UDP QGC ==
  data : Inport
  Bus Selector : BusSelector  OutputSignals=data,length
  Data Type Conversion : DataTypeConversion  SaturateOnIntegerOverflow=off  RndMeth=Floor
  UDP : slrealtimeiplib/UDP Send  useHostTargetConn=on  toAddress=127.0.0.1  toPort=14550  sampleTime=-1  enableMessage=off  localPort=14551
  wires:
  Bus Selector/1 -> UDP/1  "<data>"
  Bus Selector/2 -> Data Type Conversion/1  "<length>"
  data/1 -> Bus Selector/1
  Data Type Conversion/1 -> UDP/2

== system GCS/RX/Enabled Subsystem/Enabled Subsystem/If Action Subsystem/Subsystem ==
  In1 : Inport
  Bus Creator1 : BusCreator  Inputs=16
  Demux : Demux  Outputs=16
  Selector : Selector  InputPortWidth=58  IndexOptions=Index vector (dialog)  Indices=[1:16]  OutputSizes=1
  actuators : Outport
  wires:
  In1/1 -> Selector/1
  Bus Creator1/1 -> actuators/1  "actuators"
  Demux/1 -> Bus Creator1/1  "right_esc"
  Demux/3 -> Bus Creator1/3  "right_aileron_servo"
  Demux/2 -> Bus Creator1/2  "left_esc"
  Demux/4 -> Bus Creator1/4  "left_aileron_servo"
  Demux/5 -> Bus Creator1/5  "right_flaperon_servo"
  Demux/6 -> Bus Creator1/6  "left_flaperon_servo"
  Demux/7 -> Bus Creator1/7  "wing_tilt_servo"
  Demux/8 -> Bus Creator1/8  "parachute_servo"
  Demux/9 -> Bus Creator1/9  "right_rudder_servo"
  Demux/10 -> Bus Creator1/10  "left_rudder_servo"
  Demux/11 -> Bus Creator1/11  "right_elevator_servo"
  Demux/12 -> Bus Creator1/12  "left_elevator_servo"
  Demux/13 -> Bus Creator1/13  "tail_esc_up"
  Demux/14 -> Bus Creator1/14  "tail_esc_down"
  Demux/15 -> Bus Creator1/15  "unused15"
  Demux/16 -> Bus Creator1/16  "unused16"
  Selector/1 -> Demux/1

== system GCS/RX/Enabled Subsystem/Enabled Subsystem/If Action Subsystem/Subsystem1 ==
  In1 : Inport
  Bus Creator1 : BusCreator  Inputs=11
  Demux : Demux  Outputs=11
  Selector : Selector  InputPortWidth=58  IndexOptions=Index vector (dialog)  Indices=[(1:11) + 17]  OutputSizes=1
  Sensors : Outport
  wires:
  Selector/1 -> Demux/1
  Demux/11 -> Bus Creator1/11  "az"
  Demux/10 -> Bus Creator1/10  "ay"
  Demux/9 -> Bus Creator1/9  "ax"
  Demux/8 -> Bus Creator1/8  "VCS"
  Demux/7 -> Bus Creator1/7  "TRK"
  Demux/6 -> Bus Creator1/6  "r"
  Demux/5 -> Bus Creator1/5  "q"
  Demux/4 -> Bus Creator1/4  "p"
  Demux/2 -> Bus Creator1/2  "theta"
  Demux/3 -> Bus Creator1/3  "psi"
  Demux/1 -> Bus Creator1/1  "phi"
  Bus Creator1/1 -> Sensors/1  "Sensors"
  In1/1 -> Selector/1

== system GCS/RX/Enabled Subsystem/Enabled Subsystem/If Action Subsystem/Subsystem2 ==
  In1 : Inport
  Bus Creator1 : BusCreator  Inputs=4
  Demux : Demux
  Selector : Selector  InputPortWidth=58  IndexOptions=Index vector (dialog)  Indices=[(1:4)+29]  OutputSizes=1
  Control Inputs : Outport
  wires:
  Selector/1 -> Demux/1
  Demux/2 -> Bus Creator1/2  "pitch"
  Demux/1 -> Bus Creator1/1  "roll"
  Bus Creator1/1 -> Control Inputs/1  "Control Inputs"
  In1/1 -> Selector/1
  Demux/3 -> Bus Creator1/3  "yaw"
  Demux/4 -> Bus Creator1/4  "throttle"

== system GCS/RX/Enabled Subsystem/Enabled Subsystem/If Action Subsystem/Subsystem3 ==
  In1 : Inport
  Selector : Selector  InputPortWidth=58  IndexOptions=Index vector (dialog)  Indices=[29]  OutputSizes=1
  time : Outport
  wires:
  In1/1 -> Selector/1
  Selector/1 -> time/1  "time"

== system GCS/RX/Enabled Subsystem/Enabled Subsystem/If Action Subsystem1/Subsystem ==
  In1 : Inport
  Bus Creator1 : BusCreator  Inputs=3
  Demux : Demux  Outputs=3
  Selector : Selector  InputPortWidth=58  IndexOptions=Index vector (dialog)  Indices=[1:3]  OutputSizes=1
  EMF : Outport
  wires:
  Selector/1 -> Demux/1
  Bus Creator1/1 -> EMF/1  "EMF"
  In1/1 -> Selector/1
  Demux/2 -> Bus Creator1/2  "ulon"
  Demux/3 -> Bus Creator1/3  "udir"
  Demux/1 -> Bus Creator1/1  "ulat"

== system GCS/RX/Enabled Subsystem/Enabled Subsystem/If Action Subsystem1/Subsystem1 ==
  In1 : Inport
  Bus Creator1 : BusCreator  Inputs=2
  Demux : Demux  Outputs=2
  Selector : Selector  InputPortWidth=58  IndexOptions=Index vector (dialog)  Indices=[4,5]  OutputSizes=1
  RPM : Outport
  wires:
  Demux/1 -> Bus Creator1/1  "LPRPM"
  Demux/2 -> Bus Creator1/2  "MPRPM"
  In1/1 -> Selector/1
  Bus Creator1/1 -> RPM/1  "RPM"
  Selector/1 -> Demux/1

== system GCS/RX/Enabled Subsystem/Enabled Subsystem/If Action Subsystem1/Subsystem10 ==
  In1 : Inport
  Bus Creator1 : BusCreator  Inputs=6
  Demux : Demux  Outputs=6
  Selector : Selector  InputPortWidth=58  IndexOptions=Index vector (dialog)  Indices=[37:42]  OutputSizes=1
  NAV : Outport
  wires:
  Demux/6 -> Bus Creator1/6  "TRK_target"
  Demux/5 -> Bus Creator1/5  "DistToTarget"
  Demux/4 -> Bus Creator1/4  "WPINDEX"
  Demux/3 -> Bus Creator1/3  "SPDSIG"
  Demux/1 -> Bus Creator1/1  "LATSIG"
  Demux/2 -> Bus Creator1/2  "LONGSIG"
  In1/1 -> Selector/1
  Bus Creator1/1 -> NAV/1  "NAV"
  Selector/1 -> Demux/1

== system GCS/RX/Enabled Subsystem/Enabled Subsystem/If Action Subsystem1/Subsystem2 ==
  In1 : Inport
  Bus Creator1 : BusCreator  Inputs=6
  Demux : Demux  Outputs=6
  Selector : Selector  InputPortWidth=58  IndexOptions=Index vector (dialog)  Indices=[6:11]  OutputSizes=1
  CMDS : Outport
  wires:
  Selector/1 -> Demux/1
  Bus Creator1/1 -> CMDS/1  "CMDS"
  In1/1 -> Selector/1
  Demux/2 -> Bus Creator1/2  "PitchCmd"
  Demux/1 -> Bus Creator1/1  "phiCmd"
  Demux/3 -> Bus Creator1/3  "rCmd"
  Demux/4 -> Bus Creator1/4  "VV Cmd"
  Demux/5 -> Bus Creator1/5  "Acc Cmd"
  Demux/6 -> Bus Creator1/6  "V Cmd"

== system GCS/RX/Enabled Subsystem/Enabled Subsystem/If Action Subsystem1/Subsystem3 ==
  In1 : Inport
  Bus Creator1 : BusCreator  Inputs=6
  Demux : Demux  Outputs=6
  Selector : Selector  InputPortWidth=58  IndexOptions=Index vector (dialog)  Indices=[12:17]  OutputSizes=1
  TCS : Outport
  wires:
  Demux/6 -> Bus Creator1/6  "TWLP_Cmd/0"
  Demux/5 -> Bus Creator1/5  "TWMP_Cmd/TWCmd"
  Demux/4 -> Bus Creator1/4  "TCS Mode"
  Demux/3 -> Bus Creator1/3  "TAI/NAC/WING"
  Demux/1 -> Bus Creator1/1  "TWH"
  Demux/2 -> Bus Creator1/2  "TWV"
  In1/1 -> Selector/1
  Bus Creator1/1 -> TCS/1  "TCS"
  Selector/1 -> Demux/1

== system GCS/RX/Enabled Subsystem/Enabled Subsystem/If Action Subsystem1/Subsystem4 ==
  In1 : Inport
  Bus Creator1 : BusCreator  Inputs=8
  Demux : Demux  Outputs=8
  Selector : Selector  InputPortWidth=58  IndexOptions=Index vector (dialog)  Indices=[18:25]  OutputSizes=1
  PII : Outport
  wires:
  Selector/1 -> Demux/1
  Bus Creator1/1 -> PII/1  "PII"
  In1/1 -> Selector/1
  Demux/2 -> Bus Creator1/2  "HDGmem"
  Demux/1 -> Bus Creator1/1  "DIR"
  Demux/3 -> Bus Creator1/3  "TRKmem"
  Demux/4 -> Bus Creator1/4  "POS"
  Demux/5 -> Bus Creator1/5  "LongErr"
  Demux/6 -> Bus Creator1/6  "LatErr"
  Demux/7 -> Bus Creator1/7  "ALT"
  Demux/8 -> Bus Creator1/8  "ALTmem"

== system GCS/RX/Enabled Subsystem/Enabled Subsystem/If Action Subsystem1/Subsystem5 ==
  In1 : Inport
  Bus Creator1 : BusCreator  Inputs=7
  Demux : Demux  Outputs=7
  Selector : Selector  InputPortWidth=58  IndexOptions=Index vector (dialog)  Indices=[26:32]  OutputSizes=1
  AP : Outport
  wires:
  Demux/6 -> Bus Creator1/6  "FAP"
  Demux/5 -> Bus Creator1/5  "LND"
  Demux/4 -> Bus Creator1/4  "AXN"
  Demux/3 -> Bus Creator1/3  "NAV"
  Demux/1 -> Bus Creator1/1  "TKO"
  Demux/2 -> Bus Creator1/2  "DXN"
  In1/1 -> Selector/1
  Bus Creator1/1 -> AP/1  "AP"
  Selector/1 -> Demux/1
  Demux/7 -> Bus Creator1/7  "MANV"

== system GCS/RX/Enabled Subsystem/Enabled Subsystem/If Action Subsystem1/Subsystem6 ==
  In1 : Inport
  Bus Creator1 : BusCreator  Inputs=4
  Demux : Demux
  Selector : Selector  InputPortWidth=58  IndexOptions=Index vector (dialog)  Indices=[33:36]  OutputSizes=1
  GUIDANCE : Outport
  wires:
  Selector/1 -> Demux/1
  Bus Creator1/1 -> GUIDANCE/1  "GUIDANCE"
  In1/1 -> Selector/1
  Demux/2 -> Bus Creator1/2  "VNAV_Norm"
  Demux/1 -> Bus Creator1/1  "LNAV_Norm"
  Demux/3 -> Bus Creator1/3  "SPD_CUE"
  Demux/4 -> Bus Creator1/4  "NAV_STATUS"

== system GCS/RX/Enabled Subsystem/Enabled Subsystem/If Action Subsystem1/Subsystem7 ==
  In1 : Inport
  Bus Creator1 : BusCreator  Inputs=11
  Demux : Demux  Outputs=11
  Selector : Selector  InputPortWidth=58  IndexOptions=Index vector (dialog)  Indices=[43:53]  OutputSizes=1
  Sensors : Outport
  wires:
  Demux/6 -> Bus Creator1/6  "VLAT"
  Demux/5 -> Bus Creator1/5  "VFRD"
  Demux/4 -> Bus Creator1/4  "EAS"
  Demux/3 -> Bus Creator1/3  "hAGL"
  Demux/1 -> Bus Creator1/1  "VN"
  Demux/2 -> Bus Creator1/2  "VE"
  In1/1 -> Selector/1
  Bus Creator1/1 -> Sensors/1  "Sensors"
  Selector/1 -> Demux/1
  Demux/7 -> Bus Creator1/7  "Lat"
  Demux/8 -> Bus Creator1/8  "Long"
  Demux/9 -> Bus Creator1/9  "VV"
  Demux/10 -> Bus Creator1/10  "GC Flag"
  Demux/11 -> Bus Creator1/11  "eph"

== system GCS/RX/Enabled Subsystem/Enabled Subsystem/If Action Subsystem1/Subsystem8 ==
  In1 : Inport
  Selector : Selector  InputPortWidth=58  IndexOptions=Index vector (dialog)  Indices=[54]  OutputSizes=1
  time : Outport
  wires:
  Selector/1 -> time/1  "time"
  In1/1 -> Selector/1

== system GCS/RX/Enabled Subsystem/Enabled Subsystem/If Action Subsystem1/Subsystem9 ==
  In1 : Inport
  Bus Creator1 : BusCreator  Inputs=4
  Demux : Demux
  Selector : Selector  InputPortWidth=58  IndexOptions=Index vector (dialog)  Indices=[55:58]  OutputSizes=1
  PI : Outport
  wires:
  Demux/4 -> Bus Creator1/4  "dacc"
  Demux/3 -> Bus Creator1/3  "ddir"
  Demux/1 -> Bus Creator1/1  "dlat"
  Demux/2 -> Bus Creator1/2  "dver"
  In1/1 -> Selector/1
  Bus Creator1/1 -> PI/1  "PI"
  Selector/1 -> Demux/1

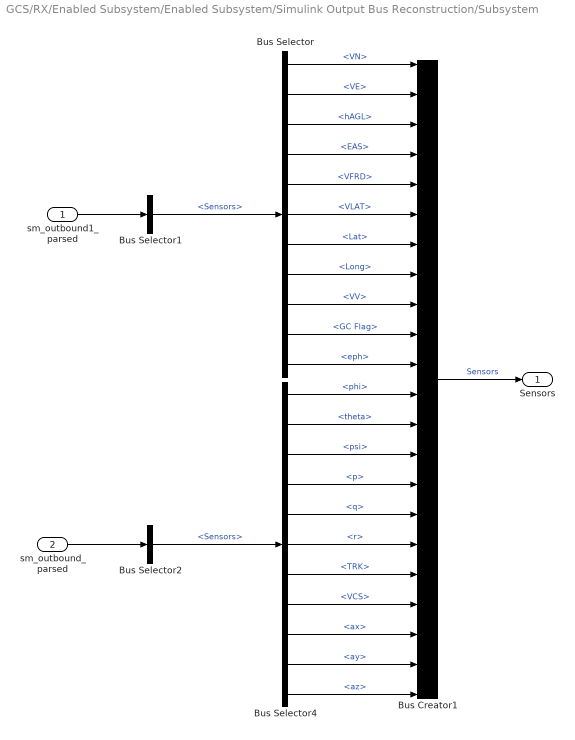
== system GCS/RX/Enabled Subsystem/Enabled Subsystem/Simulink Output Bus Reconstruction/Subsystem ==
  sm_outbound1_parsed : Inport
  sm_outbound_parsed : Inport  Port=2
  Bus Creator1 : BusCreator  Inputs=22
  Bus Selector : BusSelector  OutputSignals=VN,VE,hAGL,EAS,VFRD,VLAT,Lat,Long,VV,GC Flag,eph
  Bus Selector1 : BusSelector  OutputSignals=Sensors
  Bus Selector2 : BusSelector  OutputSignals=Sensors
  Bus Selector4 : BusSelector  OutputSignals=phi,theta,psi,p,q,r,TRK,VCS,ax,ay,az
  Sensors : Outport
  wires:
  Bus Selector/4 -> Bus Creator1/4  "<EAS>"
  Bus Selector/6 -> Bus Creator1/6  "<VLAT>"
  Bus Selector/7 -> Bus Creator1/7  "<Lat>"
  Bus Creator1/1 -> Sensors/1  "Sensors"
  Bus Selector4/5 -> Bus Creator1/16  "<q>"
  Bus Selector4/2 -> Bus Creator1/13  "<theta>"
  Bus Selector4/11 -> Bus Creator1/22  "<az>"
  Bus Selector/5 -> Bus Creator1/5  "<VFRD>"
  Bus Selector/9 -> Bus Creator1/9  "<VV>"
  Bus Selector/3 -> Bus Creator1/3  "<hAGL>"
  Bus Selector4/8 -> Bus Creator1/19  "<VCS>"
  Bus Selector/10 -> Bus Creator1/10  "<GC Flag>"
  Bus Selector/11 -> Bus Creator1/11  "<eph>"
  Bus Selector4/1 -> Bus Creator1/12  "<phi>"
  Bus Selector4/7 -> Bus Creator1/18  "<TRK>"
  Bus Selector4/4 -> Bus Creator1/15  "<p>"
  Bus Selector4/6 -> Bus Creator1/17  "<r>"
  Bus Selector/2 -> Bus Creator1/2  "<VE>"
  Bus Selector/8 -> Bus Creator1/8  "<Long>"
  Bus Selector4/3 -> Bus Creator1/14  "<psi>"
  Bus Selector4/10 -> Bus Creator1/21  "<ay>"
  Bus Selector/1 -> Bus Creator1/1  "<VN>"
  Bus Selector4/9 -> Bus Creator1/20  "<ax>"
  sm_outbound_parsed/1 -> Bus Selector2/1
  Bus Selector1/1 -> Bus Selector/1  "<Sensors>"
  sm_outbound1_parsed/1 -> Bus Selector1/1
  Bus Selector2/1 -> Bus Selector4/1  "<Sensors>"

== matlab function GCS/time since epoch ==
  data: time_s output
function time_s = fcn()
   time_s = seconds(datetime - datetime(1970,1,1,0,0,0,0));
end
